simulink model "fourch_cont"  (R2021a)
settings: Solver=VariableStepAuto  StartTime=0.0  StopTime=5  FixedStep=0.001  RelTol=1e-3
values from neighbouring files (symbols this model uses):
  A = 0.1    [four_ch.m]
  Be = 100    [four_ch.m]
  Bh = 70    [four_ch.m]
  Bm = 3.2    [four_ch.m]
  Bs = 3.2    [four_ch.m]
  Dh = 100    [four_ch.m]
  Dm = 5    [four_ch.m]
  Ds = 10    [four_ch.m]
  Fc = 1    [four_ch.m]
  Fip = 1    [four_ch.m]
  Je = 0    [four_ch.m]
  Jh = 0.5    [four_ch.m]
  Ke = 200    [four_ch.m]
  Kh = 2000    [four_ch.m]
  Km = 4    [four_ch.m]
  Ks = 4    [four_ch.m]
  Mm = 0.5    [four_ch.m]
  Ms = 2    [four_ch.m]
  Ph = 20100    [four_ch.m]
  tau = 10000    [four_ch.m]
settings Model: Creator=anuj  LastModifiedBy=antoninoparisi
settings SolverCC: AlgebraicLoopSolver=TrustRegion
settings DebuggingCC: SFMachineParentedDataDiag=warning

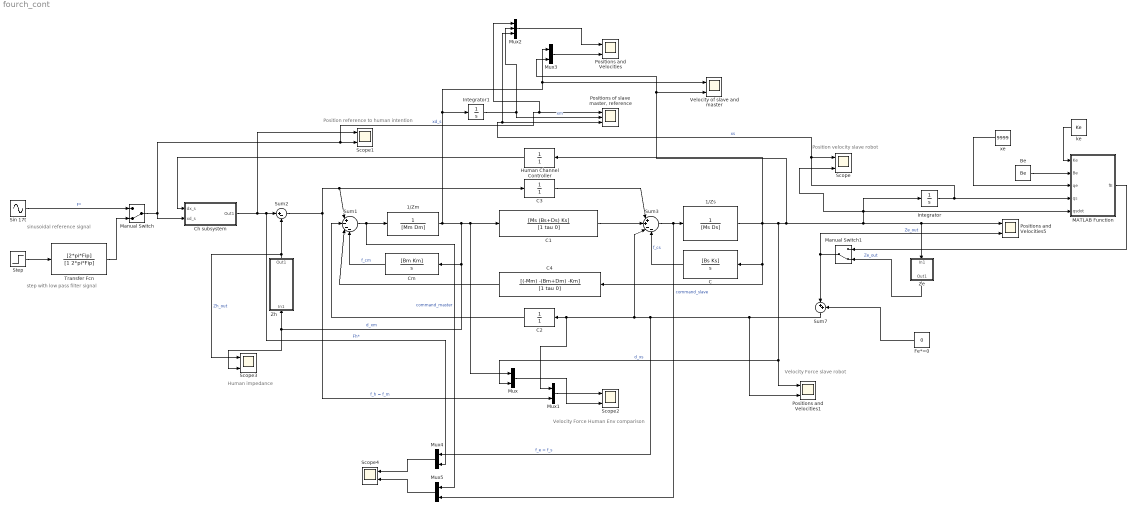
== system fourch_cont ==
  note: Human impedance
  note: Velocity Force Human Env comparison
  note: Velocity Force slave robot
  note: Position velocity slave robot
  note: sinusoidal reference signal
  note: step with low pass filter signal
  note: Position reference to human intention
  1/Zm : TransferFcn  Denominator=[Mm Dm]
  1/Zs : TransferFcn  Denominator=[Ms Ds]
  Be : Constant  Value=Be
  C : TransferFcn  Numerator=[Bs Ks]  Denominator=[1 0]
  C1 : TransferFcn  Numerator=[Ms (Bs+Ds) Ks]  Denominator=[1 tau 0]
  C2 : TransferFcn  Denominator=[1]
  C3 : TransferFcn  Denominator=[1]
  C4 : TransferFcn  Numerator=[(-Mm) -(Bm+Dm) -Km]  Denominator=[1 tau 0]
  Ch subsystem : Subsystem
  Cm : TransferFcn  Numerator=[Bm Km]  Denominator=[1 0]
  Fe*=0 : Constant  Value=0
  Human Channel Controller : TransferFcn  Denominator=[1]
  Integrator : Integrator
  Integrator1 : Integrator
  MATLAB Function : MATLAB Function  TreatAsAtomicUnit=on
  Manual Switch : ManualSwitch  CurrentSetting=0
  Manual Switch1 : ManualSwitch  CurrentSetting=0
  Mux{,1,3..5} (5 alike) : Mux  Inputs=2
  Mux2 : Mux  Inputs=3
  Positions and Velocities : Scope  NumInputPorts=2
  Positions and Velocities1 : Scope  NumInputPorts=2
  Positions and Velocities5 : Scope  NumInputPorts=2
  "Positions of slave master, reference" : Scope  NumInputPorts=3
  Scope{,1..4} (5 alike) : Scope  NumInputPorts=2
  Sin 17t : Sin  Amplitude=A  Frequency=2*pi*Fc  SampleTime=0
  Step : Step  After=A  SampleTime=0
  Sum1 : Sum  Inputs=|+---
  Sum2 : Sum  Inputs=|+-
  Sum3 : Sum  Inputs=|++--
  Sum7 : Sum  Inputs=|++
  Transfer Fcn : TransferFcn  Numerator=[2*pi*Fip]  Denominator=[1 2*pi*Fip]
  Velocity of slave and master : Scope  NumInputPorts=2
  Ze : Subsystem
  Zh : Subsystem
  ke : Constant  Value=Ke
  xe : Constant  Value=9999
  wires:
  Mux/1 -> Scope2/2
  Mux1/1 -> Scope2/1
  Sum2/1 -> Sum1/1, C3/1, Mux1/2  "f_h = f_m"
  1/Zm/1 -> Mux3/1, Velocity of slave and master/1, Integrator1/1, C1/1, Mux/1, Cm/1, Scope3/2, Zh/1(In1)  "d_xm"
  Sum1/1 -> Mux5/1, 1/Zm/1  "command_master"
  C2/1 -> Sum1/2
  C3/1 -> Sum3/1
  Sum3/1 -> Mux5/2, 1/Zs/1  "command_slave"
  Fe*=0/1 -> Sum7/2
  Sum7/1 -> Positions and Velocities1/2, Mux4/1, Sum3/3, Mux1/1, C2/1  "f_e = f_s"
  C4/1 -> Sum1/3
  Ch subsystem/1(Out1) -> Scope1/1, Mux4/2, Sum2/1  "Fh*"
  Be/1 -> MATLAB Function/2(Be)
  xe/1 -> MATLAB Function/3(qe)
  ke/1 -> MATLAB Function/1(Ke)
  Integrator/1 -> Scope/1, "Positions of slave master, reference"/3, Mux2/3, MATLAB Function/4(qs)  "xs"
  Transfer Fcn/1 -> Manual Switch/2
  Step/1 -> Transfer Fcn/1
  Human Channel Controller/1 -> Ch subsystem/1(dx_s)
  Manual Switch/1 -> Ch subsystem/2(xd_s), Mux2/1, "Positions of slave master, reference"/1, Scope1/2  "xd_s"
  Sin 17t/1 -> Manual Switch/1  "F*"
  C1/1 -> Sum3/2
  MATLAB Function/1(fE) -> Manual Switch1/1
  1/Zs/1 -> C/1, C4/1, Positions and Velocities1/1, Mux/2, Mux3/2, Velocity of slave and master/2, Scope/2, MATLAB Function/5(qsdot), Integrator/1, Positions and Velocities5/1, Ze/1(In1), Human Channel Controller/1  "d_xs"
  Manual Switch1/1 -> Positions and Velocities5/2, Sum7/1  "Ze_out"
  Zh/1(Out1) -> Scope3/1, Sum2/2  "Zh_out"
  Cm/1 -> Sum1/4  "f_cm"
  C/1 -> Sum3/4  "f_cs"
  Ze/1(Out1) -> Manual Switch1/2  "Ze_out"
  Integrator1/1 -> "Positions of slave master, reference"/2, Mux2/2  "xm"
  Mux2/1 -> Positions and Velocities/1
  Mux3/1 -> Positions and Velocities/2
  Mux4/1 -> Scope4/1
  Mux5/1 -> Scope4/2

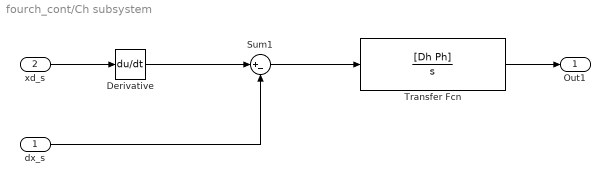
== system fourch_cont/Ch subsystem ==
  dx_s : Inport
  xd_s : Inport  Port=2
  Derivative : Derivative
  Sum1 : Sum  Inputs=|+-
  Transfer Fcn : TransferFcn  Numerator=[Dh Ph]  Denominator=[1 0]
  Out1 : Outport
  wires:
  dx_s/1 -> Sum1/2
  Sum1/1 -> Transfer Fcn/1
  xd_s/1 -> Derivative/1
  Derivative/1 -> Sum1/1
  Transfer Fcn/1 -> Out1/1

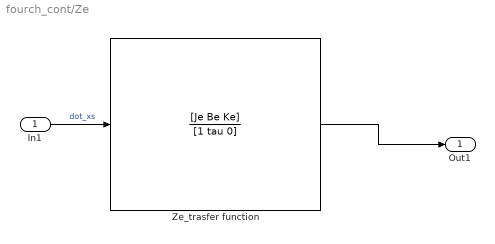
== system fourch_cont/Ze ==
  In1 : Inport
  Ze_trasfer function : TransferFcn  Numerator=[Je Be Ke]  Denominator=[1 tau 0]
  Out1 : Outport
  wires:
  In1/1 -> Ze_trasfer function/1  "dot_xs"
  Ze_trasfer function/1 -> Out1/1

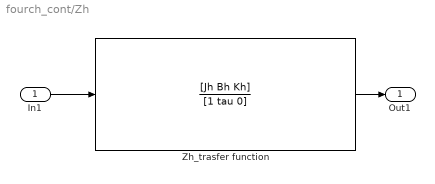
== system fourch_cont/Zh ==
  In1 : Inport
  Zh_trasfer function : TransferFcn  Numerator=[Jh Bh Kh]  Denominator=[1 tau 0]
  Out1 : Outport
  wires:
  Zh_trasfer function/1 -> Out1/1
  In1/1 -> Zh_trasfer function/1

== matlab function fourch_cont/MATLAB Function ==
  data: Ke input; fE output; Be input; qe input; qs input; qsdot input
function fE = environment(Ke, Be, qe, qs, qsdot)
    if qs > qe
        fE = Ke * (qs - qe) + Be * qsdot;
    else
        fE = 0;
    end
end
